simulink model "Event5"  (R2020b)
settings: Solver=FixedStepDiscrete  StartTime=0.0  StopTime=0.1  FixedStep=0.1  RelTol=1e-3  EnableMultiTasking=on
settings Model: Creator=BEAR  LastModifiedBy=apple
settings SolverCC: AutoInsertRateTranBlk=on
settings DataIOCC: LimitDataPoints=on  ReturnWorkspaceOutputs=off
settings OptimizationCC: LifeSpan=inf
settings DebuggingCC: AllowSymbolicDim=off  SFUnexpectedBacktrackingDiag=warning  SFNoUnconditionalDefaultTransitionDiag=warning  SFExecutionAtInitializationDiag=none  ArithmeticOperatorsInVariantConditions=warning
settings SFSimCC: SimUseLocalCustomCode=off  CustomCodeUndefinedFunction=UseInterfaceOnly
settings RTWCC: RTWUseLocalCustomCode=off
settings CodeAppCC: StateflowObjectComments=on
settings GRTTargetCC: TargetLangStandard=C89/C90 (ANSI)
settings ConfigComp: CovMetricSettings=dw  CovSaveCumulativeToWorkspaceVar=on  CovSaveSingleToWorkspaceVar=on  CovExternalEMLEnable=off  CovSFcnEnable=off

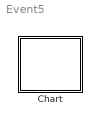
== system Event5 ==
  Chart : Stateflow chart  TreatAsAtomicUnit=on

== stateflow chart Event5/Chart ==
  state A [parallel]
    settings: executionOrder=1
    state A1
    state A2
      en: fprintf("en_A2")
    state A3
      en: fprintf("en_A3")
    (default) -> A1 : {x=-1;}
    A1 -> A2
    A2 -> A3
  state B [parallel]
    settings: executionOrder=2
    state B1
    state B2
      en: fprintf("en_B2")
    (default) -> B1
    B1 -> B2 : {fprintf("b")}/{E;fprintf("tb")}
  data: x local
  events: E local FUNCTION_CALL_EVENT; F local FUNCTION_CALL_EVENT
